simulink model "fik_gimbal"  (R2016a)
settings: Solver=VariableStepAuto  StartTime=0.0  StopTime=10.0  RelTol=1e-3
values from neighbouring files (symbols this model uses):
  A_k = -eye(3)    [transfer_ks_init.m]
  B_k = eye(3)    [transfer_ks_init.m]
  P = eye(3)    [transfer_ks_init.m]
undefined symbols (not defined in the file or in its folder): transfer_ks_init
libraries: aerolibutil x1
settings Model: Creator=glenn  LastModifiedBy=glenn
settings GRTTargetCC: GeneratePreprocessorConditionals=Use local settings

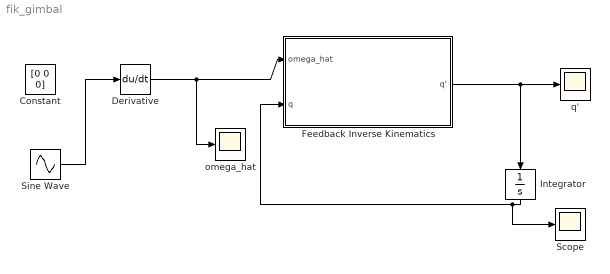
== system fik_gimbal ==
  Constant : Constant  Value=[0 0 0]
  Derivative : Derivative
  Feedback Inverse Kinematics : Subsystem
  Integrator : Integrator
  Scope : Scope
  Sine Wave : Sin  Amplitude=[1 1 1]  Phase=[0 0.5 0.8]  SampleTime=0
  omega_hat : Scope
  q' : Scope
  wires:
  Derivative/1 -> omega_hat/1, Feedback Inverse Kinematics/1(omega_hat)
  Feedback Inverse Kinematics/1(q') -> Integrator/1, q'/1
  Sine Wave/1 -> Derivative/1
  Integrator/1 -> Scope/1, Feedback Inverse Kinematics/2(q)

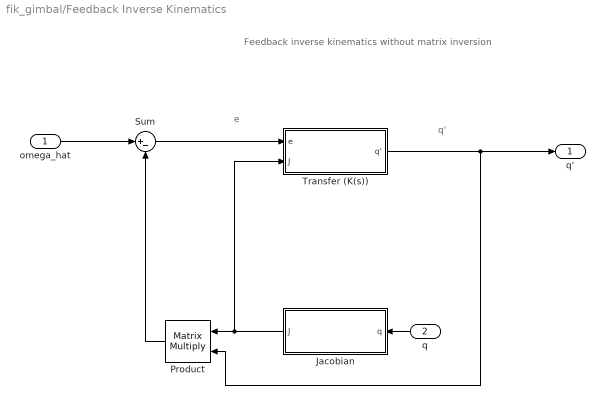
== system fik_gimbal/Feedback Inverse Kinematics ==
  note: e
  note: q'
  note: Feedback inverse kinematics without matrix inversion
  omega_hat : Inport
  q : Inport  Port=2
  Jacobian : Subsystem
  Product : Product  Multiplication=Matrix(*)
  Sum : Sum  Inputs=|+-
  Transfer (K(s)) : Subsystem  InitFcn=transfer_ks_init;
  q' : Outport
  wires:
  Jacobian/1(J) -> Product/1, Transfer (K(s))/2(J)
  omega_hat/1 -> Sum/1
  Transfer (K(s))/1(q') -> Product/2, q'/1
  Sum/1 -> Transfer (K(s))/1(e)
  q/1 -> Jacobian/1(q)
  Product/1 -> Sum/2

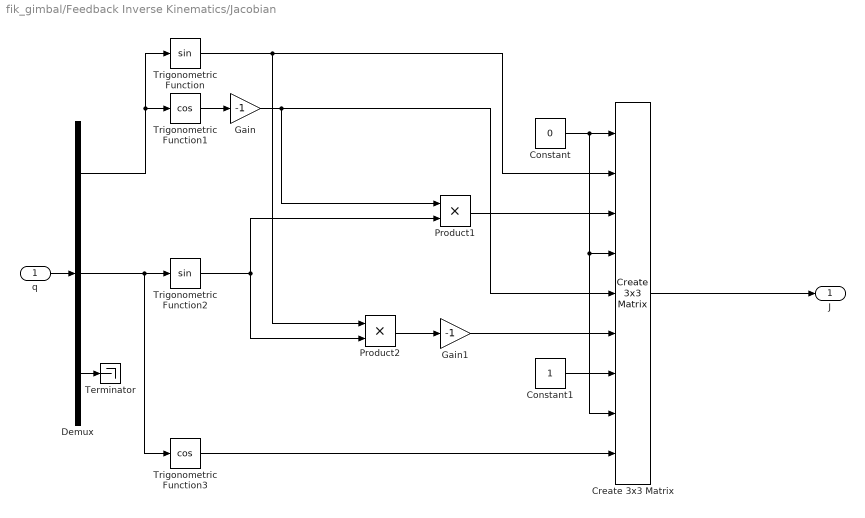
== system fik_gimbal/Feedback Inverse Kinematics/Jacobian ==
  q : Inport
  Constant : Constant  Value=0
  Constant1 : Constant
  Create 3x3 Matrix : aerolibutil/Create 3x3 Matrix
  Demux : Demux  Outputs=3
  Gain : Gain  Gain=-1
  Gain1 : Gain  Gain=-1
  Product1 : Product
  Product2 : Product
  Terminator : Terminator
  Trigonometric Function : Trigonometry
  Trigonometric Function1 : Trigonometry  Operator=cos
  Trigonometric Function2 : Trigonometry
  Trigonometric Function3 : Trigonometry  Operator=cos
  J : Outport
  wires:
  q/1 -> Demux/1
  Demux/1 -> Trigonometric Function/1, Trigonometric Function1/1
  Create 3x3 Matrix/1 -> J/1
  Constant/1 -> Create 3x3 Matrix/8, Create 3x3 Matrix/4, Create 3x3 Matrix/1
  Constant1/1 -> Create 3x3 Matrix/7
  Trigonometric Function/1 -> Product2/1, Create 3x3 Matrix/2
  Trigonometric Function1/1 -> Gain/1
  Gain/1 -> Product1/1, Create 3x3 Matrix/5
  Demux/2 -> Trigonometric Function3/1, Trigonometric Function2/1
  Trigonometric Function2/1 -> Product2/2, Product1/2
  Product1/1 -> Create 3x3 Matrix/3
  Product2/1 -> Gain1/1
  Gain1/1 -> Create 3x3 Matrix/6
  Trigonometric Function3/1 -> Create 3x3 Matrix/9
  Demux/3 -> Terminator/1

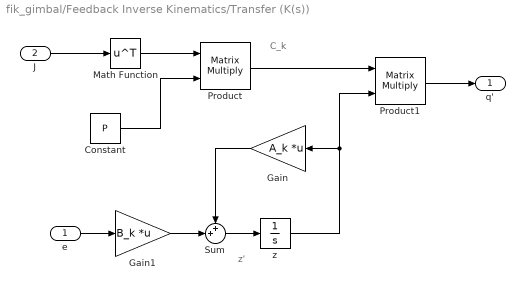
== system fik_gimbal/Feedback Inverse Kinematics/Transfer (K(s)) ==
  note: C_k
  note: z'
  e : Inport
  J : Inport  Port=2
  Constant : Constant  Value=P
  Gain : Gain  Gain=A_k  Multiplication=Matrix(K*u)
  Gain1 : Gain  Gain=B_k  Multiplication=Matrix(K*u)
  Math Function : Math  Operator=transpose  SaturateOnIntegerOverflow=on
  Product : Product  Multiplication=Matrix(*)
  Product1 : Product  Multiplication=Matrix(*)
  Sum : Sum  Inputs=++|
  z : Integrator
  q' : Outport
  wires:
  z/1 -> Gain/1, Product1/2
  Gain/1 -> Sum/1
  Sum/1 -> z/1
  e/1 -> Gain1/1
  Gain1/1 -> Sum/2
  J/1 -> Math Function/1
  Math Function/1 -> Product/1
  Constant/1 -> Product/2
  Product/1 -> Product1/1
  Product1/1 -> q'/1
